simulink model "RoboticFish_Maneuverability_model"  (R2022b)
settings: Solver=ode4  StartTime=0.0  StopTime=50  FixedStep=0.01  RelTol=1e-3  EnableMultiTasking=on
libraries: sharedutil x15, matrix_library x1, dspvision x1, vrlib x1
(part 3 of 3)

== matlab function RoboticFish_Maneuverability_model/ALL SCOPE/ESO/fal(e,0.5,h) ==
  data: u input; y output
function y = fcn(u)
%#codegen 非线性函数fal(x,α,d)
x = u(1);
alpha = u(2);
d = u(3);

if abs(x) <= d
    y = x / (d ^ (1 - alpha));
else 
    y = abs(x) ^ alpha * sign(x);
end

== matlab function RoboticFish_Maneuverability_model/ALL SCOPE/ESO2/fal(e,0.25,h) ==
  data: u input; y output
function y = fcn(u)
%#codegen 非线性函数fal(x,α,d)
x = u(1);
alpha = u(2);
d = u(3);

if abs(x) <= d
    y = x / (d ^ (1 - alpha));
else 
    y = abs(x) ^ alpha * sign(x);
end

== matlab function RoboticFish_Maneuverability_model/ALL SCOPE/ESO2/fal(e,0.5,h) ==
  data: u input; y output
function y = fcn(u)
%#codegen 非线性函数fal(x,α,d)
x = u(1);
alpha = u(2);
d = u(3);

if abs(x) <= d
    y = x / (d ^ (1 - alpha));
else 
    y = abs(x) ^ alpha * sign(x);
end

== matlab function RoboticFish_Maneuverability_model/ALL SCOPE/ESO1/fal(e,0.25,h) ==
  data: u input; y output
function y = fcn(u)
%#codegen 非线性函数fal(x,α,d)
x = u(1);
alpha = u(2);
d = u(3);

if abs(x) <= d
    y = x / (d ^ (1 - alpha));
else 
    y = abs(x) ^ alpha * sign(x);
end
